simulink model "SF042A_HwAgSnsrls"  (R2013b)
settings: Solver=FixedStepDiscrete  SolverMode=SingleTasking  StartTime=0.0  StopTime=1  FixedStep=0.002  RelTol=1e-3
values from neighbouring files (symbols this model uses):
  ARCHGLBPRM_2MILLISEC_SEC_F32 = DataDict.Constant    [SF042A_HwAgSnsrls_DataDict.m]
  CORRDPINIONAGCON_CNT_U08 = DataDict.Constant    [SF042A_HwAgSnsrls_DataDict.m]
  FCENTROFFSCON_CNT_U08 = DataDict.Constant    [SF042A_HwAgSnsrls_DataDict.m]
  HwAgSnsrlsCorrdPinionAgHwConf = DataDict.Calibration    [SF042A_HwAgSnsrls_DataDict.m]
  HwAgSnsrlsFCentrHwConf = DataDict.Calibration    [SF042A_HwAgSnsrls_DataDict.m]
  HwAgSnsrlsSmotngCoeff = DataDict.Calibration    [SF042A_HwAgSnsrls_DataDict.m]
  HwAgSnsrlsSmotngStepThd = DataDict.Calibration    [SF042A_HwAgSnsrls_DataDict.m]
  HwAgSnsrlsStordPinionConf = DataDict.Calibration    [SF042A_HwAgSnsrls_DataDict.m]
  HwAgSnsrlsStordPinionConfThd = DataDict.Calibration    [SF042A_HwAgSnsrls_DataDict.m]
  HwAgSnsrlsVehDynDifThd = DataDict.Calibration    [SF042A_HwAgSnsrls_DataDict.m]
  HwAgSnsrlsVehDynHwConf = DataDict.Calibration    [SF042A_HwAgSnsrls_DataDict.m]
  HwAgSnsrlsVehDynMotVelThd = DataDict.Calibration    [SF042A_HwAgSnsrls_DataDict.m]
  HwAgSnsrlsVehDynPinionTqThd = DataDict.Calibration    [SF042A_HwAgSnsrls_DataDict.m]
  HwAgSnsrlsVehDynTmr1Thd = DataDict.Calibration    [SF042A_HwAgSnsrls_DataDict.m]
  HwAgSnsrlsVehDynTmr2Thd = DataDict.Calibration    [SF042A_HwAgSnsrls_DataDict.m]
  HwAgSnsrlsVehDynVehSpdThd = DataDict.Calibration    [SF042A_HwAgSnsrls_DataDict.m]
  HwAgSnsrlsVehDynYawRateThd = DataDict.Calibration    [SF042A_HwAgSnsrls_DataDict.m]
  HwAgSnsrlsWhlFrqThd = DataDict.Calibration    [SF042A_HwAgSnsrls_DataDict.m]
  HwAgSnsrlsWhlSpdHwAgCoeff1 = DataDict.Calibration    [SF042A_HwAgSnsrls_DataDict.m]
  HwAgSnsrlsWhlSpdHwAgCoeff2 = DataDict.Calibration    [SF042A_HwAgSnsrls_DataDict.m]
  HwAgSnsrlsWhlSpdHwAgThd = DataDict.Calibration    [SF042A_HwAgSnsrls_DataDict.m]
  HwAgSnsrlsWhlSpdHwConf = DataDict.Calibration    [SF042A_HwAgSnsrls_DataDict.m]
  HwAgSnsrlsWhlSpdRatThd = DataDict.Calibration    [SF042A_HwAgSnsrls_DataDict.m]
  HwAgSnsrlsWhlSpdTmrThd = DataDict.Calibration    [SF042A_HwAgSnsrls_DataDict.m]
  HwAgSnsrlsWhlSpdVehSpdThd = DataDict.Calibration    [SF042A_HwAgSnsrls_DataDict.m]
  LASTPOSNCON_CNT_U08 = DataDict.Constant    [SF042A_HwAgSnsrls_DataDict.m]
  MILLISECTO100MICROSEC_ULS_U32 = DataDict.Constant    [SF042A_HwAgSnsrls_DataDict.m]
  SysGlbPrmSysKineRat = DataDict.ImprtdCal    [SF042A_HwAgSnsrls_DataDict.m]
  SysGlbPrmSysTqRat = DataDict.ImprtdCal    [SF042A_HwAgSnsrls_DataDict.m]
  VEHDYNCON_CNT_U08 = DataDict.Constant    [SF042A_HwAgSnsrls_DataDict.m]
  WHLSPDCON_CNT_U08 = DataDict.Constant    [SF042A_HwAgSnsrls_DataDict.m]
undefined symbols (not defined in the file or in its folder): NtcNr1, SigQlfr1
libraries: NxtrAbslt x11, Fil x8, NxtrLim x4, simulink x3, NxtrNvM x1, FixdToFloat x1
(part 4 of 6)

== system SF042A_HwAgSnsrls/HwAgSnsrls/HwAgSnsrlsPer1/Arbitrator/MaxHwConf/If Action Subsystem5 ==
  WhlSpdHwConf : Inport
  Action Port : ActionPort  ActionType=then
  Constant1 : Constant  Value=WHLSPDCON_CNT_U08
  CopyRight2 : Subsystem  Description=|  mask(Copyright Information){none=on}
      | Copyright info block.                                               
      |                                                                     
      | Place copyright information at the top of every subsystem in design.
      mask prompts: none "No parameters"
      mask help: Place copyright information at the top of every subsystem in design.
      mask Display:
      | NxtrConf = 'Nexteer Confidential';
      | 
      | sys = bdroot; %handle for the current model ("system")
      | first = get_param(sys,'Created');
      | if(isempty(first))
      |     first = datestr(now,'yyyy');
      | else
      |     first = first(end-3:end);  %year is last four digits
      | end
      | 
      | last = get_param(sys,'LastModifiedDate');
      | if isempty(last)
      |     last = datestr(now,'yyyy');
      | else
      |     last = last(end-3:end);
      | end
      | 
      | if strcmp(first,last)
      |     fprintf('%s -- Copyright %s Nexteer',NxtrConf,first)
      | else
      |     fprintf('%s -- %s%s- %s Nexteer',NxtrConf,char(169),first,last)
      | end
  MaxHwConf2 : Outport
  SelnCaseSt2 : Outport  Port=2
  wires:
  Constant1/1 -> SelnCaseSt2/1
  WhlSpdHwConf/1 -> MaxHwConf2/1

== system SF042A_HwAgSnsrls/HwAgSnsrls/HwAgSnsrlsPer1/Arbitrator/MaxHwConf/If Action Subsystem6 ==
  Action Port : ActionPort  ActionType=then
  Constant2 : Constant  Value=CORRDPINIONAGCON_CNT_U08
  CopyRight2 : Subsystem  Description=|  mask(Copyright Information){none=on}
      | Copyright info block.                                               
      |                                                                     
      | Place copyright information at the top of every subsystem in design.
      mask prompts: none "No parameters"
      mask help: Place copyright information at the top of every subsystem in design.
      mask Display:
      | NxtrConf = 'Nexteer Confidential';
      | 
      | sys = bdroot; %handle for the current model ("system")
      | first = get_param(sys,'Created');
      | if(isempty(first))
      |     first = datestr(now,'yyyy');
      | else
      |     first = first(end-3:end);  %year is last four digits
      | end
      | 
      | last = get_param(sys,'LastModifiedDate');
      | if isempty(last)
      |     last = datestr(now,'yyyy');
      | else
      |     last = last(end-3:end);
      | end
      | 
      | if strcmp(first,last)
      |     fprintf('%s -- Copyright %s Nexteer',NxtrConf,first)
      | else
      |     fprintf('%s -- %s%s- %s Nexteer',NxtrConf,char(169),first,last)
      | end
  Data Store Read1 : DataStoreRead  RequirementInfo={} %GIDa_b331d1ea_0b11_4856_aa2b_b39adada7baf  DataStoreName=CorrdPinionAgHwConf
  MaxHwConf : Outport
  SelnCaseSt : Outport  Port=2
  wires:
  Constant2/1 -> SelnCaseSt/1
  Data Store Read1/1 -> MaxHwConf/1

== system SF042A_HwAgSnsrls/HwAgSnsrls/HwAgSnsrlsPer1/Arbitrator/MaxHwConf/If Action Subsystem7 ==
  MaxHwConf3 : Inport
  SelnCaseSt3 : Inport  Port=2
  Action Port : ActionPort  ActionType=else
  CopyRight2 : Subsystem  Description=|  mask(Copyright Information){none=on}
      | Copyright info block.                                               
      |                                                                     
      | Place copyright information at the top of every subsystem in design.
      mask prompts: none "No parameters"
      mask help: Place copyright information at the top of every subsystem in design.
      mask Display:
      | NxtrConf = 'Nexteer Confidential';
      | 
      | sys = bdroot; %handle for the current model ("system")
      | first = get_param(sys,'Created');
      | if(isempty(first))
      |     first = datestr(now,'yyyy');
      | else
      |     first = first(end-3:end);  %year is last four digits
      | end
      | 
      | last = get_param(sys,'LastModifiedDate');
      | if isempty(last)
      |     last = datestr(now,'yyyy');
      | else
      |     last = last(end-3:end);
      | end
      | 
      | if strcmp(first,last)
      |     fprintf('%s -- Copyright %s Nexteer',NxtrConf,first)
      | else
      |     fprintf('%s -- %s%s- %s Nexteer',NxtrConf,char(169),first,last)
      | end
  MaxHwConf : Outport
  SelnCaseSt : Outport  Port=2
  wires:
  SelnCaseSt3/1 -> SelnCaseSt/1
  MaxHwConf3/1 -> MaxHwConf/1

== system SF042A_HwAgSnsrls/HwAgSnsrls/HwAgSnsrlsPer1/Arbitrator/NewHwAgConf/CopyRight2 ==

== system SF042A_HwAgSnsrls/HwAgSnsrls/HwAgSnsrlsPer1/Arbitrator/NewHwAgConf/HwAgOffsSeln ==
  note: Case 0: Forced Cneter
      | Case 1: Vehicle Dynamic
      | Case 2: Wheel Speed
      | Case 3: Stored Last Position
      | default: Corrected Pinion Angle
  StordHwAgOffs : Inport
  SelnCaseSt : Inport  Port=2
  CopyRight2 : Subsystem  Description=|  mask(Copyright Information){none=on}
      | Copyright info block.                                               
      |                                                                     
      | Place copyright information at the top of every subsystem in design.
      mask prompts: none "No parameters"
      mask help: Place copyright information at the top of every subsystem in design.
      mask Display:
      | NxtrConf = 'Nexteer Confidential';
      | 
      | sys = bdroot; %handle for the current model ("system")
      | first = get_param(sys,'Created');
      | if(isempty(first))
      |     first = datestr(now,'yyyy');
      | else
      |     first = first(end-3:end);  %year is last four digits
      | end
      | 
      | last = get_param(sys,'LastModifiedDate');
      | if isempty(last)
      |     last = datestr(now,'yyyy');
      | else
      |     last = last(end-3:end);
      | end
      | 
      | if strcmp(first,last)
      |     fprintf('%s -- Copyright %s Nexteer',NxtrConf,first)
      | else
      |     fprintf('%s -- %s%s- %s Nexteer',NxtrConf,char(169),first,last)
      | end
  CorrectedPinionAg : Subsystem  TreatAsAtomicUnit=on
  ForcedCenter : Subsystem  TreatAsAtomicUnit=on
  Merge : Merge  Inputs=5
  StordLastPosn : Subsystem  TreatAsAtomicUnit=on
  Switch Case : SwitchCase  CaseConditions={0,1,2, 3}
  VehicleDynamic : Subsystem  TreatAsAtomicUnit=on
  WheelSpeed : Subsystem  TreatAsAtomicUnit=on
  HwAgOffs : Outport
  wires:
  SelnCaseSt/1 -> Switch Case/1
  Switch Case/1 -> ForcedCenter/Action
  Switch Case/2 -> VehicleDynamic/Action
  Switch Case/3 -> WheelSpeed/Action
  Switch Case/5 -> CorrectedPinionAg/Action
  StordHwAgOffs/1 -> StordLastPosn/1(StordHwAgOffs)
  ForcedCenter/1(HwAgOffs) -> Merge/1
  VehicleDynamic/1(HwAgOffs) -> Merge/2
  WheelSpeed/1(HwAgOffs) -> Merge/3
  Switch Case/4 -> StordLastPosn/Action
  Merge/1 -> HwAgOffs/1
  StordLastPosn/1(HwAgOffs) -> Merge/4
  CorrectedPinionAg/1(HwAgOffs) -> Merge/5

== system SF042A_HwAgSnsrls/HwAgSnsrls/HwAgSnsrlsPer1/Arbitrator/PrevHwAgConf/CopyRight2 ==

== system SF042A_HwAgSnsrls/HwAgSnsrls/HwAgSnsrlsPer1/FCentr/If Action Subsystem/CopyRight2 ==

== system SF042A_HwAgSnsrls/HwAgSnsrls/HwAgSnsrlsPer1/RelHwAgCalcn/Set to 0/CopyRight2 ==

== system SF042A_HwAgSnsrls/HwAgSnsrls/HwAgSnsrlsPer1/RelHwAgCalcn/UseMotAg/CopyRight2 ==

== system SF042A_HwAgSnsrls/HwAgSnsrls/HwAgSnsrlsPer1/RelHwAgCalcn/UseMotAg/GetMotAgOffs ==
  In1 : Inport
  Action Port : ActionPort  ActionType=then
  Constant1 : Constant  RequirementInfo={} %GIDa_43157458_f2f4_4cb5_b19f_3b89b9974c5e  Value=0  OutDataTypeStr=boolean
      settings: AttributesFormatString=%<OutDataTypeStr>
  CopyRight2 : Subsystem  Description=|  mask(Copyright Information){none=on}
      | Copyright info block.                                               
      |                                                                     
      | Place copyright information at the top of every subsystem in design.
      mask prompts: none "No parameters"
      mask help: Place copyright information at the top of every subsystem in design.
      mask Display:
      | NxtrConf = 'Nexteer Confidential';
      | 
      | sys = bdroot; %handle for the current model ("system")
      | first = get_param(sys,'Created');
      | if(isempty(first))
      |     first = datestr(now,'yyyy');
      | else
      |     first = first(end-3:end);  %year is last four digits
      | end
      | 
      | last = get_param(sys,'LastModifiedDate');
      | if isempty(last)
      |     last = datestr(now,'yyyy');
      | else
      |     last = last(end-3:end);
      | end
      | 
      | if strcmp(first,last)
      |     fprintf('%s -- Copyright %s Nexteer',NxtrConf,first)
      | else
      |     fprintf('%s -- %s%s- %s Nexteer',NxtrConf,char(169),first,last)
      | end
  Data Store Write1 : DataStoreWrite  RequirementInfo={} %GIDa_2db1c057_a211_43b3_ba5c_0b69edcee649  DataStoreName=MotAgOffsEna
  Data Store Write2 : DataStoreWrite  RequirementInfo={} %GIDa_f4127d35_126c_4b0f_8986_55b94a7b93f6  DataStoreName=MotAgOffs
  wires:
  In1/1 -> Data Store Write2/1
  Constant1/1 -> Data Store Write1/1

== system SF042A_HwAgSnsrls/HwAgSnsrls/HwAgSnsrlsPer1/Smoothing/If Action Subsystem/CopyRight2 ==

== system SF042A_HwAgSnsrls/HwAgSnsrls/HwAgSnsrlsPer1/Smoothing/If Action Subsystem1/CopyRight2 ==

== system SF042A_HwAgSnsrls/HwAgSnsrls/HwAgSnsrlsPer1/VehDynAutoCentr/LpFilOne/CopyRight2 ==

== system SF042A_HwAgSnsrls/HwAgSnsrls/HwAgSnsrlsPer1/VehDynAutoCentr/LpFilOne/If Action Subsystem1 ==
  Action Port : ActionPort  ActionType=else
  CopyRight2 : Subsystem  Description=|  mask(Copyright Information){none=on}
      | Copyright info block.                                               
      |                                                                     
      | Place copyright information at the top of every subsystem in design.
      mask prompts: none "No parameters"
      mask help: Place copyright information at the top of every subsystem in design.
      mask Display:
      | NxtrConf = 'Nexteer Confidential';
      | 
      | sys = bdroot; %handle for the current model ("system")
      | first = get_param(sys,'Created');
      | if(isempty(first))
      |     first = datestr(now,'yyyy');
      | else
      |     first = first(end-3:end);  %year is last four digits
      | end
      | 
      | last = get_param(sys,'LastModifiedDate');
      | if isempty(last)
      |     last = datestr(now,'yyyy');
      | else
      |     last = last(end-3:end);
      | end
      | 
      | if strcmp(first,last)
      |     fprintf('%s -- Copyright %s Nexteer',NxtrConf,first)
      | else
      |     fprintf('%s -- %s%s- %s Nexteer',NxtrConf,char(169),first,last)
      | end
  Data Store Read : DataStoreRead  DataStoreName=PrevFildRelHwAg1
  FildRelHwAg1 : Outport
  wires:
  Data Store Read/1 -> FildRelHwAg1/1

== system SF042A_HwAgSnsrls/HwAgSnsrls/HwAgSnsrlsPer1/VehDynAutoCentr/LpFilOne/If Action Subsystem2 ==
  RelHwAg : Inport
  Action Port : ActionPort  ActionType=then
  CopyRight2 : Subsystem  Description=|  mask(Copyright Information){none=on}
      | Copyright info block.                                               
      |                                                                     
      | Place copyright information at the top of every subsystem in design.
      mask prompts: none "No parameters"
      mask help: Place copyright information at the top of every subsystem in design.
      mask Display:
      | NxtrConf = 'Nexteer Confidential';
      | 
      | sys = bdroot; %handle for the current model ("system")
      | first = get_param(sys,'Created');
      | if(isempty(first))
      |     first = datestr(now,'yyyy');
      | else
      |     first = first(end-3:end);  %year is last four digits
      | end
      | 
      | last = get_param(sys,'LastModifiedDate');
      | if isempty(last)
      |     last = datestr(now,'yyyy');
      | else
      |     last = last(end-3:end);
      | end
      | 
      | if strcmp(first,last)
      |     fprintf('%s -- Copyright %s Nexteer',NxtrConf,first)
      | else
      |     fprintf('%s -- %s%s- %s Nexteer',NxtrConf,char(169),first,last)
      | end
  FilLpUpdOutp : Fil/FilLpUpdOutp  StVar=RelHwAgFil1
      settings: AttributesFormatString=StVar: %<StVar>
  FildRelHwAg1 : Outport
  wires:
  FilLpUpdOutp/1 -> FildRelHwAg1/1
  RelHwAg/1 -> FilLpUpdOutp/1

== system SF042A_HwAgSnsrls/HwAgSnsrls/HwAgSnsrlsPer1/VehDynAutoCentr/LpFilOneEna/CopyRight2 ==

== system SF042A_HwAgSnsrls/HwAgSnsrls/HwAgSnsrlsPer1/VehDynAutoCentr/LpFilOneEna/VehDynTmr1 ==
  RelHwAg : Inport
  VehDynTmr1Ena : Inport  Port=2
  Constant1 : Constant  RequirementInfo={'linktype_rmi_doors' '00012961 (/E-STEER Core/SubSystem Specifications/Application Functions - EA4/SF042A Handwheel Angle Sensorless)' '#SF042A_74' 'true' 'REQ: SF042A_74' '' } %GIDa_85b8f9b1_07a3_4fba_948a_d116f03b650b  Value=MILLISECTO100MICROSEC_ULS_U32
  Constant3 : Constant  RequirementInfo={'linktype_rmi_doors' '00012961 (/E-STEER Core/SubSystem Specifications/Application Functions - EA4/SF042A Handwheel Angle Sensorless)' '#SF042A_74' 'true' 'REQ: SF042A_74' '' } %GIDa_cb221577_6e66_4a93_bd14_c4bcdc458cc8  Value=HwAgSnsrlsVehDynTmr1Thd
  CopyRight2 : Subsystem  Description=|  mask(Copyright Information){none=on}
      | Copyright info block.                                               
      |                                                                     
      | Place copyright information at the top of every subsystem in design.
      mask prompts: none "No parameters"
      mask help: Place copyright information at the top of every subsystem in design.
      mask Display:
      | NxtrConf = 'Nexteer Confidential';
      | 
      | sys = bdroot; %handle for the current model ("system")
      | first = get_param(sys,'Created');
      | if(isempty(first))
      |     first = datestr(now,'yyyy');
      | else
      |     first = first(end-3:end);  %year is last four digits
      | end
      | 
      | last = get_param(sys,'LastModifiedDate');
      | if isempty(last)
      |     last = datestr(now,'yyyy');
      | else
      |     last = last(end-3:end);
      | end
      | 
      | if strcmp(first,last)
      |     fprintf('%s -- Copyright %s Nexteer',NxtrConf,first)
      | else
      |     fprintf('%s -- %s%s- %s Nexteer',NxtrConf,char(169),first,last)
      | end
  Data Store Read1 : DataStoreRead  RequirementInfo={'linktype_rmi_doors' '00012961 (/E-STEER Core/SubSystem Specifications/Application Functions - EA4/SF042A Handwheel Angle Sensorless)' '#SF042A_74' 'true' 'REQ: SF042A_74' '' } %GIDa_5407714a_3970_466a_90f3_223b190911bd  DataStoreName=PrevVehDynFil1Ena
  GetTiSpan1 : Subsystem  RequirementInfo={'linktype_rmi_doors' '00012961 (/E-STEER Core/SubSystem Specifications/Application Functions - EA4/SF042A Handwheel Angle Sensorless)' '#SF042A_74' 'true' 'REQ: SF042A_74' '' } %GIDa_89e59885_3596_41af_913e_806696792d39  TreatAsAtomicUnit=on
  If : If  RequirementInfo={'linktype_rmi_doors' '00012961 (/E-STEER Core/SubSystem Specifications/Application Functions - EA4/SF042A Handwheel Angle Sensorless)' '#SF042A_74' 'true' 'REQ: SF042A_74' '' } %GIDa_39ae2832_b5f3_4118_a185_82fd1d64f369  IfExpression=u1
  If Action Subsystem3 : Subsystem  RequirementInfo={'linktype_rmi_doors' '00012961 (/E-STEER Core/SubSystem Specifications/Application Functions - EA4/SF042A Handwheel Angle Sensorless)' '#SF042A_74' 'true' 'REQ: SF042A_74' '' } %GIDa_a483e877_3d73_4c1d_bc79_73208516ba9d  TreatAsAtomicUnit=on
  If1 : If  RequirementInfo={'linktype_rmi_doors' '00012961 (/E-STEER Core/SubSystem Specifications/Application Functions - EA4/SF042A Handwheel Angle Sensorless)' '#SF042A_74' 'true' 'REQ: SF042A_74' '' } %GIDa_27d876ff_52fb_42ef_922a_1973e390179c  NumInputs=2  IfExpression=u1 & u2  ShowElse=off
  Merge : Merge  RequirementInfo={'linktype_rmi_doors' '00012961 (/E-STEER Core/SubSystem Specifications/Application Functions - EA4/SF042A Handwheel Angle Sensorless)' '#SF042A_74' 'true' 'REQ: SF042A_74' '' } %GIDa_b677e413_ab0c_487a_b637_5192dedcf434
  Product : Product  RequirementInfo={'linktype_rmi_doors' '00012961 (/E-STEER Core/SubSystem Specifications/Application Functions - EA4/SF042A Handwheel Angle Sensorless)' '#SF042A_74' 'true' 'REQ: SF042A_74' '' } %GIDa_738a14e3_97d5_45b6_b0c0_22dddeea00a6
  Relational Operator1 : RelationalOperator  RequirementInfo={'linktype_rmi_doors' '00012961 (/E-STEER Core/SubSystem Specifications/Application Functions - EA4/SF042A Handwheel Angle Sensorless)' '#SF042A_74' 'true' 'REQ: SF042A_74' '' } %GIDa_2c4f56f5_6522_4328_aa69_ad25c3e606fd  OutDataTypeStr=boolean
  Set to 0 : Subsystem  RequirementInfo={'linktype_rmi_doors' '00012961 (/E-STEER Core/SubSystem Specifications/Application Functions - EA4/SF042A Handwheel Angle Sensorless)' '#SF042A_74' 'true' 'REQ: SF042A_74' '' } %GIDa_6b67478d_6f71_4f43_8f0d_1ada5412273b  TreatAsAtomicUnit=on
  FilOneEna : Outport
  wires:
  Product/1 -> Relational Operator1/2
  Constant1/1 -> Product/2
  If/1 -> GetTiSpan1/Action
  Data Store Read1/1 -> If1/2
  If1/1 -> If Action Subsystem3/Action
  RelHwAg/1 -> If Action Subsystem3/1(RelHwAg)
  Relational Operator1/1 -> If1/1, FilOneEna/1
  Merge/1 -> Relational Operator1/1
  GetTiSpan1/1(Out1) -> Merge/1
  Constant3/1 -> Product/1
  If/2 -> Set to 0/Action
  VehDynTmr1Ena/1 -> If/1
  Set to 0/1(Out1) -> Merge/2

== system SF042A_HwAgSnsrls/HwAgSnsrls/HwAgSnsrlsPer1/VehDynAutoCentr/LpFilTwo/CopyRight2 ==

== system SF042A_HwAgSnsrls/HwAgSnsrls/HwAgSnsrlsPer1/VehDynAutoCentr/LpFilTwo/If Action Subsystem3 ==
  note: The PIM, PrevFildRelHwAg2 is removed.
      | The output, FildRelHwAg2 is removed.
  Action Port : ActionPort  ActionType=else
  Constant= : Constant  Value=0  OutDataTypeStr=single
      settings: AttributesFormatString=%<OutDataTypeStr>
  CopyRight2 : Subsystem  Description=|  mask(Copyright Information){none=on}
      | Copyright info block.                                               
      |                                                                     
      | Place copyright information at the top of every subsystem in design.
      mask prompts: none "No parameters"
      mask help: Place copyright information at the top of every subsystem in design.
      mask Display:
      | NxtrConf = 'Nexteer Confidential';
      | 
      | sys = bdroot; %handle for the current model ("system")
      | first = get_param(sys,'Created');
      | if(isempty(first))
      |     first = datestr(now,'yyyy');
      | else
      |     first = first(end-3:end);  %year is last four digits
      | end
      | 
      | last = get_param(sys,'LastModifiedDate');
      | if isempty(last)
      |     last = datestr(now,'yyyy');
      | else
      |     last = last(end-3:end);
      | end
      | 
      | if strcmp(first,last)
      |     fprintf('%s -- Copyright %s Nexteer',NxtrConf,first)
      | else
      |     fprintf('%s -- %s%s- %s Nexteer',NxtrConf,char(169),first,last)
      | end
  VehDynHwConf : Outport
  wires:
  Constant=/1 -> VehDynHwConf/1

== system SF042A_HwAgSnsrls/HwAgSnsrls/HwAgSnsrlsPer1/VehDynAutoCentr/LpFilTwo/If Action Subsystem4 ==
  RelHwAg : Inport
  Action Port : ActionPort  ActionType=then
  Constant2 : Constant  RequirementInfo={} %GIDa_8d627932_e0a7_4bbd_8cdf_a1d9eed2cdb6  Value=HwAgSnsrlsVehDynHwConf
  CopyRight2 : Subsystem  Description=|  mask(Copyright Information){none=on}
      | Copyright info block.                                               
      |                                                                     
      | Place copyright information at the top of every subsystem in design.
      mask prompts: none "No parameters"
      mask help: Place copyright information at the top of every subsystem in design.
      mask Display:
      | NxtrConf = 'Nexteer Confidential';
      | 
      | sys = bdroot; %handle for the current model ("system")
      | first = get_param(sys,'Created');
      | if(isempty(first))
      |     first = datestr(now,'yyyy');
      | else
      |     first = first(end-3:end);  %year is last four digits
      | end
      | 
      | last = get_param(sys,'LastModifiedDate');
      | if isempty(last)
      |     last = datestr(now,'yyyy');
      | else
      |     last = last(end-3:end);
      | end
      | 
      | if strcmp(first,last)
      |     fprintf('%s -- Copyright %s Nexteer',NxtrConf,first)
      | else
      |     fprintf('%s -- %s%s- %s Nexteer',NxtrConf,char(169),first,last)
      | end
  Data Store Write3 : DataStoreWrite  DataStoreName=VehDynHwAgOffs
  FilLpUpdOutp : Fil/FilLpUpdOutp  StVar=RelHwAgFil2
      settings: AttributesFormatString=StVar: %<StVar>
  VehDynHwConf : Outport
  wires:
  Constant2/1 -> VehDynHwConf/1
  FilLpUpdOutp/1 -> Data Store Write3/1
  RelHwAg/1 -> FilLpUpdOutp/1

== system SF042A_HwAgSnsrls/HwAgSnsrls/HwAgSnsrlsPer1/VehDynAutoCentr/LpFilTwoEna/CopyRight2 ==

== system SF042A_HwAgSnsrls/HwAgSnsrls/HwAgSnsrlsPer1/VehDynAutoCentr/LpFilTwoEna/VehDynTmr2 ==
  FildRelHwAg1 : Inport
  VehDynTmr2Ena : Inport  Port=2
  Constant1 : Constant  RequirementInfo={'linktype_rmi_doors' '00012961 (/E-STEER Core/SubSystem Specifications/Application Functions - EA4/SF042A Handwheel Angle Sensorless)' '#SF042A_75' 'true' 'REQ: SF042A_75' '' } %GIDa_37973adc_4458_4612_b236_81c9b07f04b3  Value=MILLISECTO100MICROSEC_ULS_U32
  Constant3 : Constant  RequirementInfo={'linktype_rmi_doors' '00012961 (/E-STEER Core/SubSystem Specifications/Application Functions - EA4/SF042A Handwheel Angle Sensorless)' '#SF042A_75' 'true' 'REQ: SF042A_75' '' } %GIDa_48941693_ea8a_4cae_9d1c_9205f9803f82  Value=HwAgSnsrlsVehDynTmr2Thd
  CopyRight2 : Subsystem  Description=|  mask(Copyright Information){none=on}
      | Copyright info block.                                               
      |                                                                     
      | Place copyright information at the top of every subsystem in design.
      mask prompts: none "No parameters"
      mask help: Place copyright information at the top of every subsystem in design.
      mask Display:
      | NxtrConf = 'Nexteer Confidential';
      | 
      | sys = bdroot; %handle for the current model ("system")
      | first = get_param(sys,'Created');
      | if(isempty(first))
      |     first = datestr(now,'yyyy');
      | else
      |     first = first(end-3:end);  %year is last four digits
      | end
      | 
      | last = get_param(sys,'LastModifiedDate');
      | if isempty(last)
      |     last = datestr(now,'yyyy');
      | else
      |     last = last(end-3:end);
      | end
      | 
      | if strcmp(first,last)
      |     fprintf('%s -- Copyright %s Nexteer',NxtrConf,first)
      | else
      |     fprintf('%s -- %s%s- %s Nexteer',NxtrConf,char(169),first,last)
      | end
  Data Store Read1 : DataStoreRead  RequirementInfo={'linktype_rmi_doors' '00012961 (/E-STEER Core/SubSystem Specifications/Application Functions - EA4/SF042A Handwheel Angle Sensorless)' '#SF042A_75' 'true' 'REQ: SF042A_75' '' } %GIDa_137ed8c6_9bd9_42e3_a32c_02f47544b6c4  DataStoreName=PrevVehDynFil2Ena
  GetTiSpan2 : Subsystem  RequirementInfo={'linktype_rmi_doors' '00012961 (/E-STEER Core/SubSystem Specifications/Application Functions - EA4/SF042A Handwheel Angle Sensorless)' '#SF042A_75' 'true' 'REQ: SF042A_75' '' } %GIDa_ff04e405_f854_456e_b9f6_876f0bc25dc6  TreatAsAtomicUnit=on
  If : If  RequirementInfo={'linktype_rmi_doors' '00012961 (/E-STEER Core/SubSystem Specifications/Application Functions - EA4/SF042A Handwheel Angle Sensorless)' '#SF042A_75' 'true' 'REQ: SF042A_75' '' } %GIDa_468fc57d_9741_46f8_9cc2_da751fddaa47  IfExpression=u1
  If Action Subsystem4 : Subsystem  RequirementInfo={'linktype_rmi_doors' '00012961 (/E-STEER Core/SubSystem Specifications/Application Functions - EA4/SF042A Handwheel Angle Sensorless)' '#SF042A_75' 'true' 'REQ: SF042A_75' '' } %GIDa_0e218ecb_d6c8_4e5d_a4a6_324a08ec560c  TreatAsAtomicUnit=on
  If1 : If  RequirementInfo={'linktype_rmi_doors' '00012961 (/E-STEER Core/SubSystem Specifications/Application Functions - EA4/SF042A Handwheel Angle Sensorless)' '#SF042A_75' 'true' 'REQ: SF042A_75' '' } %GIDa_a47e3fd2_ab88_4d56_b91e_c9945ffca385  NumInputs=2  IfExpression=u1 & u2  ShowElse=off
  Merge : Merge  RequirementInfo={'linktype_rmi_doors' '00012961 (/E-STEER Core/SubSystem Specifications/Application Functions - EA4/SF042A Handwheel Angle Sensorless)' '#SF042A_75' 'true' 'REQ: SF042A_75' '' } %GIDa_8e369bd4_b560_4017_99b4_f5ff52e6cb15
  Product : Product  RequirementInfo={'linktype_rmi_doors' '00012961 (/E-STEER Core/SubSystem Specifications/Application Functions - EA4/SF042A Handwheel Angle Sensorless)' '#SF042A_75' 'true' 'REQ: SF042A_75' '' } %GIDa_cd24f930_3b67_4c4f_ab91_583fb24bbe24
  Relational Operator1 : RelationalOperator  RequirementInfo={'linktype_rmi_doors' '00012961 (/E-STEER Core/SubSystem Specifications/Application Functions - EA4/SF042A Handwheel Angle Sensorless)' '#SF042A_75' 'true' 'REQ: SF042A_75' '' } %GIDa_9247e66e_ff25_4569_ac1b_745d89e94d7d  OutDataTypeStr=boolean
  Set to 0 : Subsystem  RequirementInfo={'linktype_rmi_doors' '00012961 (/E-STEER Core/SubSystem Specifications/Application Functions - EA4/SF042A Handwheel Angle Sensorless)' '#SF042A_75' 'true' 'REQ: SF042A_75' '' } %GIDa_aba40a15_4988_45f7_81df_3cd88798262a  TreatAsAtomicUnit=on
  FilTwoEna : Outport
  wires:
  Product/1 -> Relational Operator1/2
  Constant1/1 -> Product/2
  Data Store Read1/1 -> If1/2
  If1/1 -> If Action Subsystem4/Action
  FildRelHwAg1/1 -> If Action Subsystem4/1(FildRelHwAg1)
  Relational Operator1/1 -> FilTwoEna/1, If1/1
  Merge/1 -> Relational Operator1/1
  GetTiSpan2/1(Out1) -> Merge/1
  Constant3/1 -> Product/1
  If/1 -> GetTiSpan2/Action
  If/2 -> Set to 0/Action
  VehDynTmr2Ena/1 -> If/1
  Set to 0/1(Out1) -> Merge/2

== system SF042A_HwAgSnsrls/HwAgSnsrls/HwAgSnsrlsPer1/VehDynAutoCentr/PinionTqCalc/CopyRight2 ==

== system SF042A_HwAgSnsrls/HwAgSnsrls/HwAgSnsrlsPer1/WhlSpdAutoCentr/WhlFrqNotVld/CopyRight2 ==

== system SF042A_HwAgSnsrls/HwAgSnsrls/HwAgSnsrlsPer1/WhlSpdAutoCentr/WhlSpd/CopyRight2 ==

== system SF042A_HwAgSnsrls/HwAgSnsrls/HwAgSnsrlsPer1/WhlSpdAutoCentr/WhlSpd/If Action Subsystem ==
  note: Use (WhlLeFrq - WhlRiFrq)/ (WhlLeFrq + WhlRiFrq)
  WhlRiFrq : Inport
  WhlLeFrq : Inport  Port=2
  Action Port : ActionPort  ActionType=then
  Add : Sum  RequirementInfo={'linktype_rmi_doors' '00012961 (/E-STEER Core/SubSystem Specifications/Application Functions - EA4/SF042A Handwheel Angle Sensorless)' '#SF042A_65' 'true' 'REQ: SF042A_65' '' } %GIDa_84d4d30b_d356_4207_894b_d03082b35a21  Inputs=+-
  Add1 : Sum  RequirementInfo={'linktype_rmi_doors' '00012961 (/E-STEER Core/SubSystem Specifications/Application Functions - EA4/SF042A Handwheel Angle Sensorless)' '#SF042A_65' 'true' 'REQ: SF042A_65' '' } %GIDa_39a5a002_951c_4bd6_88d8_f991d6d2b67e
  CopyRight2 : Subsystem  Description=|  mask(Copyright Information){none=on}
      | Copyright info block.                                               
      |                                                                     
      | Place copyright information at the top of every subsystem in design.
      mask prompts: none "No parameters"
      mask help: Place copyright information at the top of every subsystem in design.
      mask Display:
      | NxtrConf = 'Nexteer Confidential';
      | 
      | sys = bdroot; %handle for the current model ("system")
      | first = get_param(sys,'Created');
      | if(isempty(first))
      |     first = datestr(now,'yyyy');
      | else
      |     first = first(end-3:end);  %year is last four digits
      | end
      | 
      | last = get_param(sys,'LastModifiedDate');
      | if isempty(last)
      |     last = datestr(now,'yyyy');
      | else
      |     last = last(end-3:end);
      | end
      | 
      | if strcmp(first,last)
      |     fprintf('%s -- Copyright %s Nexteer',NxtrConf,first)
      | else
      |     fprintf('%s -- %s%s- %s Nexteer',NxtrConf,char(169),first,last)
      | end
  Divide : Product  RequirementInfo={'linktype_rmi_doors' '00012961 (/E-STEER Core/SubSystem Specifications/Application Functions - EA4/SF042A Handwheel Angle Sensorless)' '#SF042A_65' 'true' 'REQ: SF042A_65' '' } %GIDa_2847553e_7fb2_4fc1_bafa_886143e285de  Inputs=*/
  WhlSpdRat : Outport
  wires:
  WhlLeFrq/1 -> Add1/1, Add/1
  WhlRiFrq/1 -> Add1/2, Add/2
  Add1/1 -> Divide/2
  Add/1 -> Divide/1
  Divide/1 -> WhlSpdRat/1

== system SF042A_HwAgSnsrls/HwAgSnsrls/HwAgSnsrlsPer1/WhlSpdAutoCentr/WhlSpd/If Action Subsystem1 ==
  note: HwAgSnsrlsWhlSpdHwAgCoeff2 is used for inventing, and may
      | be removed in the future.
  WhlSpdRat : Inport
  RelHwAg : Inport  Port=2
  Action Port : ActionPort  ActionType=then
  Abslt_f32_f1 : NxtrAbslt/Abslt_f32_f32  RequirementInfo={'linktype_rmi_doors' '00012961 (/E-STEER Core/SubSystem Specifications/Application Functions - EA4/SF042A Handwheel Angle Sensorless)' '#SF042A_70' 'true' 'REQ: SF042A_70' '' } %GIDa_8b98395d_120d_4408_a26e_88da54c890e9  SFunctionSpec=single y1 = Abslt_f32_f32(single u1)
      settings: AttributesFormatString=%<Name>
  Add1 : Sum  RequirementInfo={'linktype_rmi_doors' '00012961 (/E-STEER Core/SubSystem Specifications/Application Functions - EA4/SF042A Handwheel Angle Sensorless)' '#SF042A_70' 'true' 'REQ: SF042A_70' '' } %GIDa_692094a2_e82b_4055_83e0_ff77edd80f35
  Constant2 : Constant  RequirementInfo={'linktype_rmi_doors' '00012961 (/E-STEER Core/SubSystem Specifications/Application Functions - EA4/SF042A Handwheel Angle Sensorless)' '#SF042A_70' 'true' 'REQ: SF042A_70' '' } %GIDa_dcbfa998_0b30_4403_b52c_0b6358551198  Value=HwAgSnsrlsWhlSpdHwAgCoeff1
  Constant3 : Constant  RequirementInfo={'linktype_rmi_doors' '00012961 (/E-STEER Core/SubSystem Specifications/Application Functions - EA4/SF042A Handwheel Angle Sensorless)' '#SF042A_70' 'true' 'REQ: SF042A_70' '' } %GIDa_9142f618_c1d5_418d_b036_5cfae17b6a9c  Value=HwAgSnsrlsWhlSpdHwAgCoeff2
  Constant4 : Constant  RequirementInfo={'linktype_rmi_doors' '00012961 (/E-STEER Core/SubSystem Specifications/Application Functions - EA4/SF042A Handwheel Angle Sensorless)' '#SF042A_70' 'true' 'REQ: SF042A_70' '' } %GIDa_aa16daa2_ae03_4fb3_8394_80112292ee4b  Value=HwAgSnsrlsWhlSpdHwAgThd
  CopyRight2 : Subsystem  Description=|  mask(Copyright Information){none=on}
      | Copyright info block.                                               
      |                                                                     
      | Place copyright information at the top of every subsystem in design.
      mask prompts: none "No parameters"
      mask help: Place copyright information at the top of every subsystem in design.
      mask Display:
      | NxtrConf = 'Nexteer Confidential';
      | 
      | sys = bdroot; %handle for the current model ("system")
      | first = get_param(sys,'Created');
      | if(isempty(first))
      |     first = datestr(now,'yyyy');
      | else
      |     first = first(end-3:end);  %year is last four digits
      | end
      | 
      | last = get_param(sys,'LastModifiedDate');
      | if isempty(last)
      |     last = datestr(now,'yyyy');
      | else
      |     last = last(end-3:end);
      | end
      | 
      | if strcmp(first,last)
      |     fprintf('%s -- Copyright %s Nexteer',NxtrConf,first)
      | else
      |     fprintf('%s -- %s%s- %s Nexteer',NxtrConf,char(169),first,last)
      | end
  If Action Subsystem3 : Subsystem  RequirementInfo={'linktype_rmi_doors' '00012961 (/E-STEER Core/SubSystem Specifications/Application Functions - EA4/SF042A Handwheel Angle Sensorless)' '#SF042A_70' 'true' 'REQ: SF042A_70' '' } %GIDa_221441a7_1ea2_4de6_84fa_de9862995654  TreatAsAtomicUnit=on
  If2 : If  RequirementInfo={'linktype_rmi_doors' '00012961 (/E-STEER Core/SubSystem Specifications/Application Functions - EA4/SF042A Handwheel Angle Sensorless)' '#SF042A_70' 'true' 'REQ: SF042A_70' '' } %GIDa_7715f038_dded_4d8d_8693_bde7e167246a  IfExpression=u1  ShowElse=off
  Product : Product  RequirementInfo={'linktype_rmi_doors' '00012961 (/E-STEER Core/SubSystem Specifications/Application Functions - EA4/SF042A Handwheel Angle Sensorless)' '#SF042A_70' 'true' 'REQ: SF042A_70' '' } %GIDa_2a2d99c0_e011_431a_b878_25fb636e963e
  Relational Operator2 : RelationalOperator  RequirementInfo={'linktype_rmi_doors' '00012961 (/E-STEER Core/SubSystem Specifications/Application Functions - EA4/SF042A Handwheel Angle Sensorless)' '#SF042A_70' 'true' 'REQ: SF042A_70' '' } %GIDa_e824dcb3_f09e_4774_9204_29066f28f443  Operator=<=  OutDataTypeStr=boolean
  wires:
  RelHwAg/1 -> If Action Subsystem3/2(RelHwAg)
  [WhlSpdCalcdHwAg] -> If Action Subsystem3/1(WhlSpdCalcdHwAg)
  If2/1 -> If Action Subsystem3/Action
  WhlSpdRat/1 -> Product/1
  Constant2/1 -> Product/2
  Constant3/1 -> Add1/2
  Product/1 -> Add1/1
  Add1/1 -> [WhlSpdCalcdHwAg], Abslt_f32_f1/1
  Constant4/1 -> Relational Operator2/2
  Abslt_f32_f1/1 -> Relational Operator2/1
  Relational Operator2/1 -> If2/1

== system SF042A_HwAgSnsrls/HwAgSnsrls/HwAgSnsrlsPer1/WhlSpdAutoCentr/WhlSpd/Output 0 ==
  Action Port : ActionPort  ActionType=else
  Constant : Constant  RequirementInfo={'linktype_rmi_doors' '00012961 (/E-STEER Core/SubSystem Specifications/Application Functions - EA4/SF042A Handwheel Angle Sensorless)' '#SF042A_65' 'true' 'REQ: SF042A_65' '' } %GIDa_0eb66ac8_95cb_4ca6_9ac5_905155561a6c  Value=0  OutDataTypeStr=single
      settings: AttributesFormatString=%<OutDataTypeStr>
  CopyRight2 : Subsystem  Description=|  mask(Copyright Information){none=on}
      | Copyright info block.                                               
      |                                                                     
      | Place copyright information at the top of every subsystem in design.
      mask prompts: none "No parameters"
      mask help: Place copyright information at the top of every subsystem in design.
      mask Display:
      | NxtrConf = 'Nexteer Confidential';
      | 
      | sys = bdroot; %handle for the current model ("system")
      | first = get_param(sys,'Created');
      | if(isempty(first))
      |     first = datestr(now,'yyyy');
      | else
      |     first = first(end-3:end);  %year is last four digits
      | end
      | 
      | last = get_param(sys,'LastModifiedDate');
      | if isempty(last)
      |     last = datestr(now,'yyyy');
      | else
      |     last = last(end-3:end);
      | end
      | 
      | if strcmp(first,last)
      |     fprintf('%s -- Copyright %s Nexteer',NxtrConf,first)
      | else
      |     fprintf('%s -- %s%s- %s Nexteer',NxtrConf,char(169),first,last)
      | end
  WhlSpdRat : Outport
  wires:
  Constant/1 -> WhlSpdRat/1

== system SF042A_HwAgSnsrls/HwAgSnsrls/HwAgSnsrlsPer1/WhlSpdAutoCentr/WhlSpd/VehSpdChk ==
  VehSpd : Inport
  Abslt_f32_f3 : NxtrAbslt/Abslt_f32_f32  RequirementInfo={'linktype_rmi_doors' '00012961 (/E-STEER Core/SubSystem Specifications/Application Functions - EA4/SF042A Handwheel Angle Sensorless)' '#SF042A_70' 'true' 'REQ: SF042A_70' '' } %GIDa_07f6f7db_005f_47ca_8384_aa092e9e8b8e  SFunctionSpec=single y1 = Abslt_f32_f32(single u1)
      settings: AttributesFormatString=%<Name>
  Constant1 : Constant  RequirementInfo={'linktype_rmi_doors' '00012961 (/E-STEER Core/SubSystem Specifications/Application Functions - EA4/SF042A Handwheel Angle Sensorless)' '#SF042A_70' 'true' 'REQ: SF042A_70' '' } %GIDa_741f4542_958f_4968_8868_4d021982ac9c  Value=MILLISECTO100MICROSEC_ULS_U32
  Constant3 : Constant  RequirementInfo={'linktype_rmi_doors' '00012961 (/E-STEER Core/SubSystem Specifications/Application Functions - EA4/SF042A Handwheel Angle Sensorless)' '#SF042A_70' 'true' 'REQ: SF042A_70' '' } %GIDa_821b1036_ebba_45ee_84ec_0d79049376a8  Value=HwAgSnsrlsWhlSpdVehSpdThd
  Constant4 : Constant  RequirementInfo={'linktype_rmi_doors' '00012961 (/E-STEER Core/SubSystem Specifications/Application Functions - EA4/SF042A Handwheel Angle Sensorless)' '#SF042A_70' 'true' 'REQ: SF042A_70' '' } %GIDa_b879748b_9070_4b1e_ac6e_ea45f7664d21  Value=HwAgSnsrlsWhlSpdTmrThd
  CopyRight2 : Subsystem  Description=|  mask(Copyright Information){none=on}
      | Copyright info block.                                               
      |                                                                     
      | Place copyright information at the top of every subsystem in design.
      mask prompts: none "No parameters"
      mask help: Place copyright information at the top of every subsystem in design.
      mask Display:
      | NxtrConf = 'Nexteer Confidential';
      | 
      | sys = bdroot; %handle for the current model ("system")
      | first = get_param(sys,'Created');
      | if(isempty(first))
      |     first = datestr(now,'yyyy');
      | else
      |     first = first(end-3:end);  %year is last four digits
      | end
      | 
      | last = get_param(sys,'LastModifiedDate');
      | if isempty(last)
      |     last = datestr(now,'yyyy');
      | else
      |     last = last(end-3:end);
      | end
      | 
      | if strcmp(first,last)
      |     fprintf('%s -- Copyright %s Nexteer',NxtrConf,first)
      | else
      |     fprintf('%s -- %s%s- %s Nexteer',NxtrConf,char(169),first,last)
      | end
  "GetTiSpan " : Subsystem  RequirementInfo={'linktype_rmi_doors' '00012961 (/E-STEER Core/SubSystem Specifications/Application Functions - EA4/SF042A Handwheel Angle Sensorless)' '#SF042A_70' 'true' 'REQ: SF042A_70' '' } %GIDa_19ad992b_c9eb_4237_af10_acfecefc6363  TreatAsAtomicUnit=on
  If2 : If  RequirementInfo={'linktype_rmi_doors' '00012961 (/E-STEER Core/SubSystem Specifications/Application Functions - EA4/SF042A Handwheel Angle Sensorless)' '#SF042A_70' 'true' 'REQ: SF042A_70' '' } %GIDa_cbd521d4_f436_442a_ae1e_34ab21b2a872  IfExpression=u1
  Merge1 : Merge  RequirementInfo={'linktype_rmi_doors' '00012961 (/E-STEER Core/SubSystem Specifications/Application Functions - EA4/SF042A Handwheel Angle Sensorless)' '#SF042A_70' 'true' 'REQ: SF042A_70' '' } %GIDa_f164b641_56da_4ef7_9853_547059c05b83
  Product : Product  RequirementInfo={'linktype_rmi_doors' '00012961 (/E-STEER Core/SubSystem Specifications/Application Functions - EA4/SF042A Handwheel Angle Sensorless)' '#SF042A_70' 'true' 'REQ: SF042A_70' '' } %GIDa_f10b513e_1901_44e3_9f4f_32972ed9ec57
  Relational Operator4 : RelationalOperator  RequirementInfo={'linktype_rmi_doors' '00012961 (/E-STEER Core/SubSystem Specifications/Application Functions - EA4/SF042A Handwheel Angle Sensorless)' '#SF042A_70' 'true' 'REQ: SF042A_70' '' } %GIDa_fe79a950_1aef_44a8_ad36_475fb219af70  OutDataTypeStr=boolean
  Relational Operator5 : RelationalOperator  RequirementInfo={'linktype_rmi_doors' '00012961 (/E-STEER Core/SubSystem Specifications/Application Functions - EA4/SF042A Handwheel Angle Sensorless)' '#SF042A_70' 'true' 'REQ: SF042A_70' '' } %GIDa_2ad7e696_f358_4731_8499_c4749387c223  OutDataTypeStr=boolean
  Set to 0 : Subsystem  RequirementInfo={'linktype_rmi_doors' '00012961 (/E-STEER Core/SubSystem Specifications/Application Functions - EA4/SF042A Handwheel Angle Sensorless)' '#SF042A_70' 'true' 'REQ: SF042A_70' '' } %GIDa_8136710d_8ad3_460c_9284_6796804d94d0  TreatAsAtomicUnit=on
  WhlSpdVehSpdEna : Outport
  wires:
  Product/1 -> Relational Operator5/2
  Constant1/1 -> Product/2
  If2/2 -> Set to 0/Action
  "GetTiSpan "/1(Out1) -> Merge1/1
  Merge1/1 -> Relational Operator5/1
  Constant4/1 -> Product/1
  Set to 0/1(Out1) -> Merge1/2
  Relational Operator5/1 -> WhlSpdVehSpdEna/1
  Constant3/1 -> Relational Operator4/2
  Abslt_f32_f3/1 -> Relational Operator4/1
  Relational Operator4/1 -> If2/1
  VehSpd/1 -> Abslt_f32_f3/1
  If2/1 -> "GetTiSpan "/Action

== system SF042A_HwAgSnsrls/HwAgSnsrls/HwAgSnsrlsPer1/Arbitrator/MaxHwConf/If Action Subsystem/CopyRight2 ==

== system SF042A_HwAgSnsrls/HwAgSnsrls/HwAgSnsrlsPer1/Arbitrator/MaxHwConf/If Action Subsystem1/CopyRight2 ==

== system SF042A_HwAgSnsrls/HwAgSnsrls/HwAgSnsrlsPer1/Arbitrator/MaxHwConf/If Action Subsystem2/CopyRight2 ==

== system SF042A_HwAgSnsrls/HwAgSnsrls/HwAgSnsrlsPer1/Arbitrator/MaxHwConf/If Action Subsystem3/CopyRight2 ==

== system SF042A_HwAgSnsrls/HwAgSnsrls/HwAgSnsrlsPer1/Arbitrator/MaxHwConf/If Action Subsystem4/CopyRight2 ==

== system SF042A_HwAgSnsrls/HwAgSnsrls/HwAgSnsrlsPer1/Arbitrator/MaxHwConf/If Action Subsystem5/CopyRight2 ==

== system SF042A_HwAgSnsrls/HwAgSnsrls/HwAgSnsrlsPer1/Arbitrator/MaxHwConf/If Action Subsystem6/CopyRight2 ==

== system SF042A_HwAgSnsrls/HwAgSnsrls/HwAgSnsrlsPer1/Arbitrator/MaxHwConf/If Action Subsystem7/CopyRight2 ==

== system SF042A_HwAgSnsrls/HwAgSnsrls/HwAgSnsrlsPer1/Arbitrator/NewHwAgConf/HwAgOffsSeln/CopyRight2 ==

== system SF042A_HwAgSnsrls/HwAgSnsrls/HwAgSnsrlsPer1/Arbitrator/NewHwAgConf/HwAgOffsSeln/CorrectedPinionAg ==
  Action Port : ActionPort  ActionType=default
  CopyRight2 : Subsystem  Description=|  mask(Copyright Information){none=on}
      | Copyright info block.                                               
      |                                                                     
      | Place copyright information at the top of every subsystem in design.
      mask prompts: none "No parameters"
      mask help: Place copyright information at the top of every subsystem in design.
      mask Display:
      | NxtrConf = 'Nexteer Confidential';
      | 
      | sys = bdroot; %handle for the current model ("system")
      | first = get_param(sys,'Created');
      | if(isempty(first))
      |     first = datestr(now,'yyyy');
      | else
      |     first = first(end-3:end);  %year is last four digits
      | end
      | 
      | last = get_param(sys,'LastModifiedDate');
      | if isempty(last)
      |     last = datestr(now,'yyyy');
      | else
      |     last = last(end-3:end);
      | end
      | 
      | if strcmp(first,last)
      |     fprintf('%s -- Copyright %s Nexteer',NxtrConf,first)
      | else
      |     fprintf('%s -- %s%s- %s Nexteer',NxtrConf,char(169),first,last)
      | end
  Data Store Read1 : DataStoreRead  DataStoreName=CorrdPinionAgHwAgOffs
  HwAgOffs : Outport
  wires:
  Data Store Read1/1 -> HwAgOffs/1

== system SF042A_HwAgSnsrls/HwAgSnsrls/HwAgSnsrlsPer1/Arbitrator/NewHwAgConf/HwAgOffsSeln/ForcedCenter ==
  Action Port : ActionPort  ActionType=case
  CopyRight2 : Subsystem  Description=|  mask(Copyright Information){none=on}
      | Copyright info block.                                               
      |                                                                     
      | Place copyright information at the top of every subsystem in design.
      mask prompts: none "No parameters"
      mask help: Place copyright information at the top of every subsystem in design.
      mask Display:
      | NxtrConf = 'Nexteer Confidential';
      | 
      | sys = bdroot; %handle for the current model ("system")
      | first = get_param(sys,'Created');
      | if(isempty(first))
      |     first = datestr(now,'yyyy');
      | else
      |     first = first(end-3:end);  %year is last four digits
      | end
      | 
      | last = get_param(sys,'LastModifiedDate');
      | if isempty(last)
      |     last = datestr(now,'yyyy');
      | else
      |     last = last(end-3:end);
      | end
      | 
      | if strcmp(first,last)
      |     fprintf('%s -- Copyright %s Nexteer',NxtrConf,first)
      | else
      |     fprintf('%s -- %s%s- %s Nexteer',NxtrConf,char(169),first,last)
      | end
  Data Store Read4 : DataStoreRead  RequirementInfo={} %GIDa_ee4faa74_31b7_40fc_8a09_b41fdcb53913  DataStoreName=FCentrHwAgOffs
  HwAgOffs : Outport
  wires:
  Data Store Read4/1 -> HwAgOffs/1

== system SF042A_HwAgSnsrls/HwAgSnsrls/HwAgSnsrlsPer1/Arbitrator/NewHwAgConf/HwAgOffsSeln/StordLastPosn ==
  StordHwAgOffs : Inport
  Action Port : ActionPort  ActionType=case
  CopyRight2 : Subsystem  Description=|  mask(Copyright Information){none=on}
      | Copyright info block.                                               
      |                                                                     
      | Place copyright information at the top of every subsystem in design.
      mask prompts: none "No parameters"
      mask help: Place copyright information at the top of every subsystem in design.
      mask Display:
      | NxtrConf = 'Nexteer Confidential';
      | 
      | sys = bdroot; %handle for the current model ("system")
      | first = get_param(sys,'Created');
      | if(isempty(first))
      |     first = datestr(now,'yyyy');
      | else
      |     first = first(end-3:end);  %year is last four digits
      | end
      | 
      | last = get_param(sys,'LastModifiedDate');
      | if isempty(last)
      |     last = datestr(now,'yyyy');
      | else
      |     last = last(end-3:end);
      | end
      | 
      | if strcmp(first,last)
      |     fprintf('%s -- Copyright %s Nexteer',NxtrConf,first)
      | else
      |     fprintf('%s -- %s%s- %s Nexteer',NxtrConf,char(169),first,last)
      | end
  HwAgOffs : Outport
  wires:
  StordHwAgOffs/1 -> HwAgOffs/1

== system SF042A_HwAgSnsrls/HwAgSnsrls/HwAgSnsrlsPer1/Arbitrator/NewHwAgConf/HwAgOffsSeln/VehicleDynamic ==
  Action Port : ActionPort  ActionType=case
  CopyRight2 : Subsystem  Description=|  mask(Copyright Information){none=on}
      | Copyright info block.                                               
      |                                                                     
      | Place copyright information at the top of every subsystem in design.
      mask prompts: none "No parameters"
      mask help: Place copyright information at the top of every subsystem in design.
      mask Display:
      | NxtrConf = 'Nexteer Confidential';
      | 
      | sys = bdroot; %handle for the current model ("system")
      | first = get_param(sys,'Created');
      | if(isempty(first))
      |     first = datestr(now,'yyyy');
      | else
      |     first = first(end-3:end);  %year is last four digits
      | end
      | 
      | last = get_param(sys,'LastModifiedDate');
      | if isempty(last)
      |     last = datestr(now,'yyyy');
      | else
      |     last = last(end-3:end);
      | end
      | 
      | if strcmp(first,last)
      |     fprintf('%s -- Copyright %s Nexteer',NxtrConf,first)
      | else
      |     fprintf('%s -- %s%s- %s Nexteer',NxtrConf,char(169),first,last)
      | end
  Data Store Read2 : DataStoreRead  DataStoreName=VehDynHwAgOffs
  HwAgOffs : Outport
  wires:
  Data Store Read2/1 -> HwAgOffs/1
